simulink model "mcb_pmsm_foc_sensorless_f28379d"  (R2023b)
settings: Solver=FixedStepDiscrete  StartTime=0.0  StopTime=6  FixedStep=Auto  RelTol=1e-3  EnableMultiTasking=on
InitFcn:
  | mcb_pmsm_foc_sensorless_f28379d_datascript;
model workspace (MAT data in the model file):
  encoderResolution = 2000
  hallOffset = '0.5'
  indexOffset = 850
  polePairs = '4'
values from neighbouring files (symbols this model uses):
  acceleration = 0.5/Ts_speed/PU_System.N_base    [mcb_pmsm_foc_sensorless_f28379d_datascript.m]
  dataType = 'single'    [mcb_pmsm_foc_sensorless_f28379d_datascript.m]    (also in mcb_pmsm_foc_test_f28379d_data.m)
  inverter = mcb_updateInverterParameters(pmsm,inverter,target)    [mcb_pmsm_foc_sensorless_f28379d_datascript.m]    (also in mcb_pmsm_foc_test_f28379d_data.m)
  PI_params = mcb_SetControllerParameters(pmsm,inverter,PU_System,T_pwm,2*Ts,Ts_speed)    [mcb_pmsm_foc_sensorless_f28379d_datascript.m]    (also in mcb_pmsm_foc_test_f28379d_data.m = mcb_SetControllerParameters(pmsm,inverter,PU_System,T_pwm,Ts)
  pmsm = mcb_SetPMSMMotorParameters("new")    [mcb_pmsm_foc_sensorless_f28379d_datascript.m]    (also in mcb_pmsm_foc_test_f28379d_data.m = mcb_SetPMSMMotorParameters("SF2804"))
  PU_System = mcb_SetPUSystem(pmsm,inverter)    [mcb_pmsm_foc_sensorless_f28379d_datascript.m]    (also in mcb_pmsm_foc_test_f28379d_data.m)
  Speed_openLoop_PU = 0.1    [mcb_pmsm_foc_sensorless_f28379d_datascript.m]
  T = Ts    (= 5e-05)    [mcb_pmsm_foc_sensorless_f28379d_datascript.m]
  T_Ref_openLoop = 1    [mcb_pmsm_foc_sensorless_f28379d_datascript.m]
  target = mcb_SetProcessorDetails('F28379D',PWM_frequency)    [mcb_pmsm_foc_sensorless_f28379d_datascript.m]    (also in mcb_pmsm_foc_test_f28379d_data.m)
  Ts = T_pwm    [discrete_tansfer_fcn.m]    (also in mcb_pmsm_foc_sensorless_f28379d_datascript.m = 5e-05; mcb_pmsm_foc_test_f28379d_data.m = 5e-05)
  Ts_motor = T_pwm/2    (= 2.5e-05)    [mcb_pmsm_foc_sensorless_f28379d_datascript.m]    (also in mcb_pmsm_foc_test_f28379d_data.m)
  Ts_sensor = 20*Ts    (= 0.001)    [mcb_pmsm_foc_sensorless_f28379d_datascript.m]    (also in mcb_pmsm_foc_test_f28379d_data.m; virtual_speed.m)
  Ts_simulink = T_pwm/2    (= 2.5e-05)    [mcb_pmsm_foc_sensorless_f28379d_datascript.m]    (also in mcb_pmsm_foc_test_f28379d_data.m)
  Ts_speed = 20*Ts    (= 0.001)    [mcb_pmsm_foc_sensorless_f28379d_datascript.m]    (also in mcb_pmsm_foc_test_f28379d_data.m = 0.0005)
undefined symbols (not defined in the file or in its folder): DiscIntNeverNeededParam, Down, GPTRIP1SEL, GPTRIP2SEL, TZ1, TZ2, Up
libraries: mcbcontrolslib x13, simulink x12, c2802xlib x7, mcbpositiondecoderlib x5, c280xlib x5, slpidlib x4, c2837xDlib x4, mcbsensorlessestimatorlib x2, svdschedulerlib x2, svdutilitieslib x1, mcbplantlib x1, autolibpmsmexterior x1
(part 4 of 4)

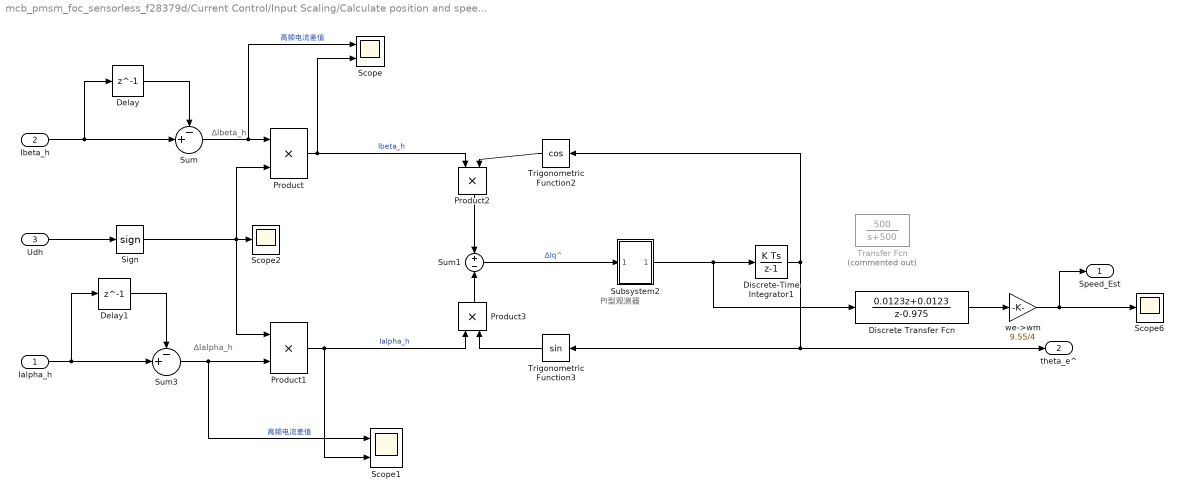
== system mcb_pmsm_foc_sensorless_f28379d/Current Control/Input Scaling/Calculate position and speed/HFI/位置和转速观测器/位置估算 ==
  note: PI型观测器
  note: ∆Ialpha_h
  note: ∆Ibeta_h
  Ialpha_h : Inport
  Ibeta_h : Inport  Port=2
  Udh : Inport  Port=3
  Delay : Delay  DelayLength=1
  Delay1 : Delay  DelayLength=1
  Discrete Transfer Fcn : DiscreteTransferFcn  Numerator=[0.0123 0.0123]  Denominator=[1 -0.975]
  Discrete-Time Integrator1 : DiscreteIntegrator  SampleTime=-1  ICPrevOutput=DiscIntNeverNeededParam  ICPrevScaledInput=DiscIntNeverNeededParam
  Product{,1..3} (4 alike) : Product
  Scope : Scope  NumInputPorts=2
  Scope1 : Scope  NumInputPorts=2
  Scope2 : Scope
  Scope6 : Scope
  Sign : Signum
  Subsystem2 : Subsystem  mask{Kp=10, Ki=25, UpperLimit=2*pi*6000/15, LowerLimit=-2*pi*6000/15}
      mask Display: disp('PI')
  Sum : Sum  Inputs=-+|
  Sum1 : Sum  Inputs=+|-
  Sum3 : Sum  Inputs=-+|
  Transfer Fcn : TransferFcn  Commented=on  Numerator=[500]  Denominator=[1 500]
  Trigonometric Function2 : Trigonometry  Operator=cos
  Trigonometric Function3 : Trigonometry
  we->wm : Gain  Gain=9.55/4
  Speed_Est : Outport  VectorParamsAs1DForOutWhenUnconnected=off
  theta_e^ : Outport  Port=2  VectorParamsAs1DForOutWhenUnconnected=off
  wires:
  Discrete-Time Integrator1/1 -> theta_e^/1, Trigonometric Function3/1, Trigonometric Function2/1
  Trigonometric Function2/1 -> Product2/2
  Product2/1 -> Sum1/1
  Trigonometric Function3/1 -> Product3/2
  Sum1/1 -> Subsystem2/1(In1)  "∆Iq^"
  Product3/1 -> Sum1/2
  we->wm/1 -> Scope6/1, Speed_Est/1
  Ialpha_h/1 -> Sum3/2, Delay1/1
  Ibeta_h/1 -> Delay/1, Sum/2
  Delay/1 -> Sum/1
  Delay1/1 -> Sum3/1
  Product/1 -> Scope/2, Product2/1  "Ibeta_h"
  Sum/1 -> Scope/1, Product/1  "高频电流差值"
  Sum3/1 -> Scope1/1, Product1/2  "高频电流差值"
  Product1/1 -> Scope1/2, Product3/1  "Ialpha_h"
  Sign/1 -> Scope2/1, Product/2, Product1/1
  Udh/1 -> Sign/1
  Subsystem2/1(Out1) -> Discrete Transfer Fcn/1, Discrete-Time Integrator1/1
  Discrete Transfer Fcn/1 -> we->wm/1

== system mcb_pmsm_foc_sensorless_f28379d/Hardware Init/Variant Subsystem/Code Generation/Calculate ADC Offset /For Iterator Subsystem/If Action Subsystem ==
  In1 : Inport
  In2 : Inport  Port=2
  Action Port : ActionPort  ActionPortLabel=if(u1 > 8)
  Memory : Memory  InheritSampleTime=on
  Memory1 : Memory  InheritSampleTime=on
  Sum : Sum
  Sum1 : Sum
  Out1 : Outport
  Out2 : Outport  Port=2
  wires:
  In1/1 -> Sum/1
  Sum/1 -> Out1/1, Memory/1
  In2/1 -> Sum1/1
  Memory/1 -> Sum/2
  Sum1/1 -> Out2/1, Memory1/1
  Memory1/1 -> Sum1/2

== system mcb_pmsm_foc_sensorless_f28379d/Current Control/Input Scaling/Calculate position and speed/HFI/位置和转速观测器/位置估算/Subsystem2 ==
  In1 : Inport
  Add1 : Sum
  Discrete-Time Integrator1 : DiscreteIntegrator  SampleTime=-1  LimitOutput=on  UpperSaturationLimit=UpperLimit  LowerSaturationLimit=LowerLimit  ICPrevOutput=DiscIntNeverNeededParam  ICPrevScaledInput=DiscIntNeverNeededParam
  Gain : Gain  Gain=9.55/4
  Ki : Gain  Gain=Ki
  Kp : Gain  Gain=Kp
  Saturation : Saturate  UpperLimit=UpperLimit  LowerLimit=LowerLimit
  Zero-Order Hold : ZeroOrderHold  SampleTime=-1
  n_est : Scope
  Out1 : Outport  VectorParamsAs1DForOutWhenUnconnected=off
  wires:
  In1/1 -> Kp/1, Ki/1
  Ki/1 -> Discrete-Time Integrator1/1
  Zero-Order Hold/1 -> Add1/1  "Kp"
  Add1/1 -> Saturation/1
  Discrete-Time Integrator1/1 -> Gain/1, Add1/2  "Ki"
  Saturation/1 -> Out1/1
  Kp/1 -> Zero-Order Hold/1
  Gain/1 -> n_est/1

== matlab function mcb_pmsm_foc_sensorless_f28379d/Subsystem/MATLAB Function ==
  data: speed_ref_rpm input; pu output; Ts input
function pu = periodic_pu_pos(speed_ref_rpm, Ts)
% 根据参考转速生成周期变化的转子位置标幺值
% 入口：
%   speed_ref_rpm - 参考转速（rpm）
%   Ts            - 调用周期（s）
% 出口：
%   pu            - 转子位置 0~1

persistent theta
if isempty(theta), theta = 0; end

% 每拍走过的“转数”
delta = (speed_ref_rpm/60)*Ts;   % rpm -> rps -> 转/拍

theta = mod(theta + delta, 1);   % 积分并归一化
pu    = single(theta);
end

== stateflow chart mcb_pmsm_foc_sensorless_f28379d/Speed Control/PI_Controller_Speed2/Chart ==
  state IDLE
    Motor_State = 1;
  state AlignStage
    Motor_State = 2;
  state OpenStage
    Motor_State = 3;
  state RunStage
    Motor_State = 4;
  note: &&CloseLoop_Enable==true
  (default) -> IDLE
  IDLE -> AlignStage : [Motor_Enable==true]
  AlignStage -> OpenStage [order 2] : [after(1000,tick)]
  OpenStage -> RunStage [order 1] : [after(3000,tick)&&CloseLoop_Enable==true]
  OpenStage -> IDLE [order 2] : [Motor_Enable==false]
  RunStage -> IDLE : [Motor_Enable==false]
  AlignStage -> IDLE [order 1] : [Motor_Enable==false]
  data: Motor_State output uint16; Motor_Enable input; CloseLoop_Enable input

== matlab function mcb_pmsm_foc_sensorless_f28379d/Speed Control/PI_Controller_Speed2/Switch Case Action Subsystem2/Subsystem2/Subsystem/MATLAB Function ==
  data: speed_ref_rpm input; pu output; Ts input
function pu = periodic_pu_pos(speed_ref_rpm, Ts)
% 根据参考转速生成周期变化的转子位置标幺值
% 入口：
%   speed_ref_rpm - 参考转速（rpm）
%   Ts            - 调用周期（s）
% 出口：
%   pu            - 转子位置 0~1

persistent theta
if isempty(theta), theta = 0; end

% 每拍走过的“转数”
delta = (speed_ref_rpm/60)*Ts;   % rpm -> rps -> 转/拍

theta = mod(theta + delta, 1);   % 积分并归一化
pu    = single(theta);
end
